simulink model "Q1_4"  (R2023b)
settings: Solver=VariableStepAuto  StartTime=0.0  StopTime=50  FixedStep=0.001  RelTol=1e-3
libraries: mpclib x1, slpidlib x1
settings Model: Creator=sayed  LastModifiedBy=sayed

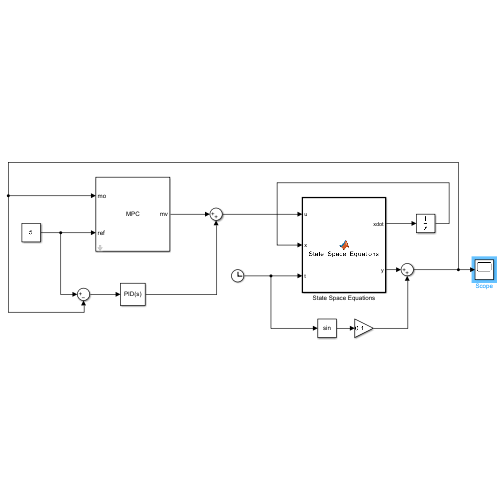
[thumbnail: Simulink's stored preview of the top-level diagram]
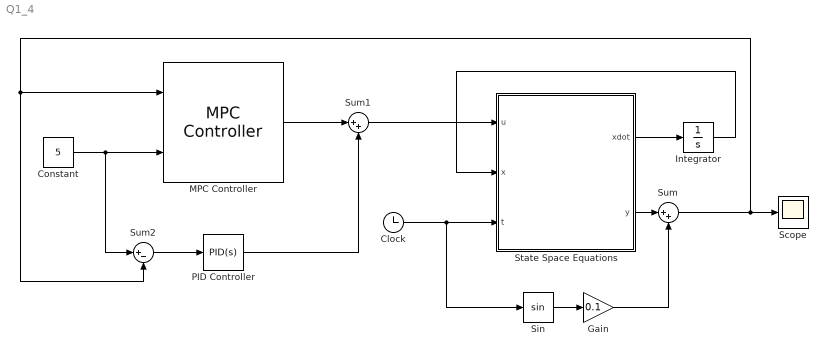
== system Q1_4 ==
  Clock : Clock
  Constant : Constant  Value=5
  Gain : Gain  Gain=0.1
  Integrator : Integrator  InitialCondition=[0;0;0;0]
  MPC Controller : mpclib/MPC Controller  SCDEnableBlockLinearizationSpecification=on  mpcobj=mpc1  is_multiple=0  enable_value=0  return_u0=off  updateMPCinCallerWorkspace=on  md_inport=off  mv_inport=off  uref_inport=off  return_cost=off  return_mvseq=off  return_qpstatus=off  return_xseq=off  return_state=off  return_ovseq=off  state_inport=off  umin_inport=off  umax_inport=off  ymin_inport=off  ymax_inport=off  cc_inport=off  ywt_inport=off  uwt_inport=off  duwt_inport=off  rhoeps_inport=off  pm_inport=off  MaximumP=10  HorizonChoice=FixedHorizon  n_ts=0.01  n_p=100  n_mv=1  n_md=0  n_ud=0  n_mo=1  n_uo=0  BlockDataType=double  SampleTimeInherited=off  switch_inport=off
  PID Controller : slpidlib/PID Controller  Controller=PID  Form=Parallel  TimeDomain=Continuous-time  UseExternalTs=off  SampleTime=-1  IntegratorMethod=Forward Euler  FilterMethod=Forward Euler  ControllerParametersSource=internal  P=25  I=15  UseKiTs=off  D=50  N=140  UseFilter=on  TunerSelectOption=Transfer Function Based (PID Tuner App)  InitialConditionSource=internal  InitialConditionForIntegrator=0  InitialConditionForFilter=0  DifferentiatorICPrevScaledInput=0  ExternalReset=none  TrackingMode=off  Kt=1  LimitOutput=off  SatLimitsSource=internal  UpperSaturationLimit=inf  LowerSaturationLimit=-inf  LinearizeAsGain=on  AntiWindupMode=none  Kb=1  LimitIntegrator=off  UpperIntegratorSaturationLimit=inf  LowerIntegratorSaturationLimit=-inf  POutMin=[]  POutMax=[]  IOutMin=[]  IOutMax=[]  DOutMin=[]  DOutMax=[]  NOutMin=[]  NOutMax=[]  SumOutMin=[]  SumOutMax=[]  SaturationOutMin=[]  SaturationOutMax=[]  PParamMin=[]  PParamMax=[]  IParamMin=[]  IParamMax=[]  DParamMin=[]  DParamMax=[]  NParamMin=[]  NParamMax=[]  KbParamMin=[]  KbParamMax=[]  KtParamMin=[]  KtParamMax=[]  KbOutMin=[]  KbOutMax=[]  KtOutMin=[]  KtOutMax=[]  IntegratorOutMin=[]  IntegratorOutMax=[]  FilterOutMin=[]  FilterOutMax=[]  SumI1OutMin=[]  SumI1OutMax=[]  SumI2OutMin=[]  SumI2OutMax=[]  SumI3OutMin=[]  SumI3OutMax=[]  SumI4OutMin=[]  SumI4OutMax=[]  SumDOutMin=[]  SumDOutMax=[]  DifferentiatorOutMin=[]  DifferentiatorOutMax=[]  FilterDiffOutCoefMin=[]  FilterDiffOutCoefMax=[]  ReciprocalOutMin=[]  ReciprocalOutMax=[]  SumDenOutMin=[]  SumDenOutMax=[]  SumNumOutMin=[]  SumNumOutMax=[]  DivideOutMin=[]  DivideOutMax=[]  UdiffTsProdOutMin=[]  UdiffTsProdOutMax=[]  NTsProdOutMin=[]  NTsProdOutMax=[]  UintegralTsProdOutMin=[]  UintegralTsProdOutMax=[]  UngainTsProdOutMin=[]  UngainTsProdOutMax=[]  ClampingZeroOutDataTypeStr=Inherit: Inherit via back propagation  ClampingZeroOutMin=[]  ClampingZeroOutMax=[]  FilterDenConstantOutDataTypeStr=Inherit: Inherit via back propagation  FilterDenConstantOutMin=[]  FilterDenConstantOutMax=[]  PCopyOutDataTypeStr=Inherit: Inherit via back propagation  PCopyOutMin=[]  PCopyOutMax=[]  NCopyOutDataTypeStr=Inherit: Inherit via back propagation  NCopyOutMin=[]  NCopyOutMax=[]  IntegratorContinuousStateAttributes=''  IntegratorStateMustResolveToSignalObject=off  IntegratorRTWStateStorageClass=Auto  FilterContinuousStateAttributes=''  FilterStateMustResolveToSignalObject=off  FilterRTWStateStorageClass=Auto  ParallelPVariant=InternalParameters  IdealPVariant=Disabled  IVariant=InternalParameters  DVariant=InternalParameters  IntegratorVariant=Continuous  SatVariant=Disabled  AWVariant=Passthrough  PCopyVariant=Disabled  TRVariant=Disabled  FdbkBlocksVariant=Forward  IdealPFdbkVariant=Disabled  SatFdbkVariant=Disabled  DerivativeFilterVariant=ContFilter  NVariant=InternalParameters  NCopyVariant=Disabled  FilterICVariant=InternalICsFilter  IntegratorICVariant=InternalICs  ExternalResetVariant=Disabled  TRSumVariant=Passthrough  SumFdbkVariant=Disabled  SumVariant=Sum_PID  TsampFilterVariant=InternalTs  TsampNgainVariant=Passthrough  TsampIntegralVariant=Disabled_SignalSpec  ExternalSaturationOutDataTypeStr=Inherit: Same as second input
  Scope : Scope
  Sin : Trigonometry
  State Space Equations : MATLAB Function  TreatAsAtomicUnit=on
  Sum : Sum  Inputs=|++
  Sum1 : Sum  Inputs=|++
  Sum2 : Sum  Inputs=|+-
  wires:
  Clock/1 -> Sin/1, State Space Equations/3(t)
  State Space Equations/1(xdot) -> Integrator/1
  Integrator/1 -> State Space Equations/2(x)
  State Space Equations/2(y) -> Sum/1
  Constant/1 -> Sum2/1, MPC Controller/2
  Sin/1 -> Gain/1
  Sum/1 -> MPC Controller/1, Sum2/2, Scope/1
  Gain/1 -> Sum/2
  MPC Controller/1 -> Sum1/1
  Sum1/1 -> State Space Equations/1(u)
  PID Controller/1 -> Sum1/2
  Sum2/1 -> PID Controller/1

== matlab function Q1_4/State Space Equations ==
  data: xdot output; u input; y output; x input; t input
function [xdot, y] = State_Space_Equations(u, x, t)

% Parameter ranges pertaining to the linear transfer function (Table 1)

ke = 75 + 25 * sin(t);
Ks = 0.375 + 0.125 * sin(t);
Kp = 2.5*10^(-12) + 2.5*10^(-12) * sin(t);
C1 = 2*10^(-11) + 1*10^(-11) * sin(t);
d = 700 + 100 * sin(t);
ma = 20.0 + 0.1 * sin(t);
Ai = 0.00203 + 0.0001 * sin(t);
Ao = 0.00152 + 0.00008 * sin(t);
ksp = 0.0012 + 0.0001 * sin(t);
tau = 35 + 5 * sin(t);

% Definig the parameters calculated for the state-space equations

a1 = (tau * (Kp * ma + C1 * d) + (C1 * ma)) / (tau * C1 * ma);
a2 = (tau * (Kp * d + C1 * ke + Ai^2 + Ao^2) + (Kp * ma + C1 * d)) / (tau * C1 * ma);
a3 = (tau * Kp * ke + Kp * d + C1 * ke + Ai^2 + Ao^2) / (tau * C1 * ma);
a4 = (Kp * ke) / (tau * C1 * ma);
beta = (ksp * Ks * ke * (Ai + Ao)) / (tau * C1 * ma);

% State-Space Matrices

A = [
    0,1,0,0;
    0,0,1,0;
    0,0,0,1;
    -a4,-a3,-a2,-a1
    ];

B = [
    0;
    0;
    0;
    beta
    ];

C = [1,0,0,0]; 

% State-Space equations

xdot = A * x + B * u;
y = C * x;
